simulink model "Project3_Trial"  (R2019a)
settings: Solver=VariableStepAuto  StartTime=0.0  StopTime=50  MaxStep=.01  RelTol=1e-3
settings Model: Creator=razue  LastModifiedBy=razue

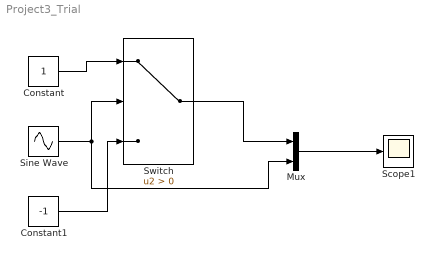
== system Project3_Trial ==
  Constant : Constant
  Constant1 : Constant  Value=-1
  Mux : Mux  Inputs=2
  Scope1 : Scope
  Sine Wave : Sin  SampleTime=0
  Switch : Switch  Criteria=u2 > Threshold
  wires:
  Sine Wave/1 -> Mux/2, Switch/2
  Constant1/1 -> Switch/3
  Constant/1 -> Switch/1
  Mux/1 -> Scope1/1
  Switch/1 -> Mux/1
